simulink model "simulation"  (R2020a)
settings: Solver=VariableStepAuto  StartTime=0.0  StopTime=50  RelTol=1e-3
libraries: SignalEditorBlockLib x3
settings Model: Creator=MILAD  LastModifiedBy=payagostar
settings DataIOCC: ReturnWorkspaceOutputs=off
settings DebuggingCC: ArithmeticOperatorsInVariantConditions=warning
settings SFSimCC: CustomCodeUndefinedFunction=UseInterfaceOnly

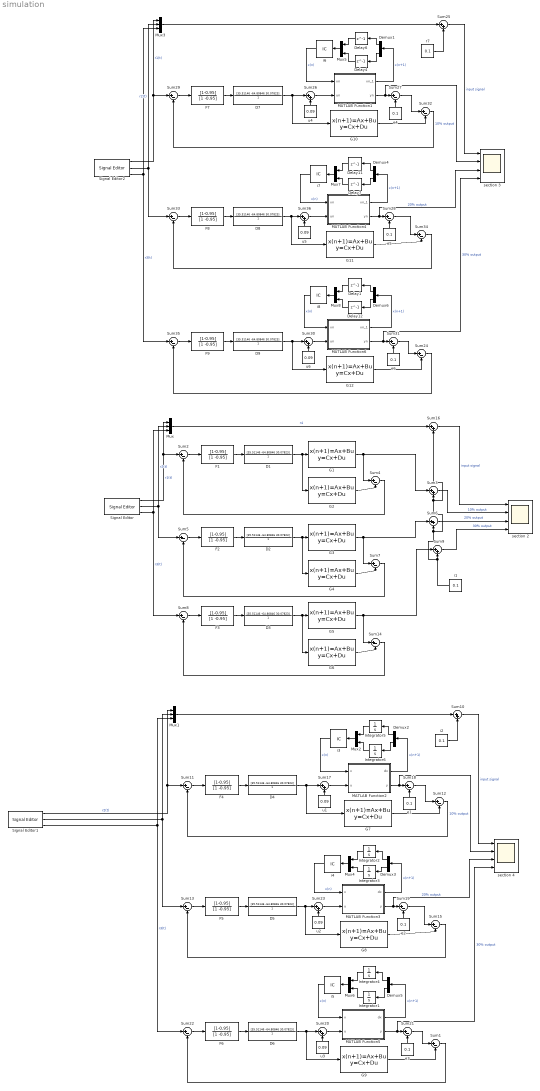
== system simulation ==
  " section 2" : Scope  NumInputPorts=4
  D{1..9} (9 alike) : DiscreteFilter  Numerator=[35.51146 -64.80846 30.07823]  Denominator=1  SampleTime=0.166
  Delay{1,4,6..7,11..12} (6 alike) : Delay  DelayLength=1  InitialCondition=0  SampleTime=0.166
  Demux{1..6} (6 alike) : Demux  Outputs=2
  F{1..9} (9 alike) : DiscreteFilter  Numerator=[1-0.95]  Denominator=[1 -0.95]  SampleTime=0.166
  G{1..12} (12 alike) : DiscreteStateSpace  A=[0.9884 0.1523;-0.1354 0.8361]  B=[0.01447;0.1693]  C=[1 0]  D=0  SampleTime=0.166
  Integrator1 : Integrator
  Integrator2 : Integrator  InitialCondition=0.1
  Integrator3 : Integrator
  Integrator4 : Integrator  InitialCondition=0.1
  Integrator5 : Integrator  InitialCondition=0.1
  Integrator6 : Integrator
  MATLAB Function1 : MATLAB Function  TreatAsAtomicUnit=on
  MATLAB Function2 : MATLAB Function  TreatAsAtomicUnit=on
  MATLAB Function3 : MATLAB Function  TreatAsAtomicUnit=on
  MATLAB Function4 : MATLAB Function  TreatAsAtomicUnit=on
  MATLAB Function5 : MATLAB Function  TreatAsAtomicUnit=on
  MATLAB Function6 : MATLAB Function  TreatAsAtomicUnit=on
  Mux : Mux  Inputs=3
  Mux1 : Mux  Inputs=3
  Mux{2,4..8} (6 alike) : Mux  Inputs=2
  Mux3 : Mux  Inputs=3
  Signal Editor : SignalEditorBlockLib/Signal Editor  FileName=r.mat  ActiveScenario=signal  ActiveSignal=Signal 3  IsBus=off  OutputBusObjectStr=Bus: BusObject  SampleTime=0.166  Interpolate=off  ZeroCross=off  OutputAfterFinalValue=Setting to zero  Unit=inherit  PreserveSignalName=on
  Signal Editor1 : SignalEditorBlockLib/Signal Editor  FileName=r.mat  ActiveScenario=signal  ActiveSignal=Signal 3  IsBus=off  OutputBusObjectStr=Bus: BusObject  SampleTime=0.166  Interpolate=off  ZeroCross=off  OutputAfterFinalValue=Setting to zero  Unit=inherit  PreserveSignalName=on
  Signal Editor2 : SignalEditorBlockLib/Signal Editor  FileName=r.mat  ActiveScenario=signal  ActiveSignal=Signal 3  IsBus=off  OutputBusObjectStr=Bus: BusObject  SampleTime=0.166  Interpolate=off  ZeroCross=off  OutputAfterFinalValue=Setting to zero  Unit=inherit  PreserveSignalName=on
  Sum{1..2,4..5,7..8,11..15,18..19,21..22,24,27..29,31..35} (24 alike) : Sum  Inputs=|+-
  Sum{3,6,9..10,16..17,20,23,25..26,30,36} (12 alike) : Sum  Inputs=|++
  e{1..6} (6 alike) : Constant  Value=0.1  SampleTime=0.166
  i1 : Constant  Value=0.1  SampleTime=0.166
  i2 : Constant  Value=0.1  SampleTime=0.166
  i{3..8} (6 alike) : InitialCondition  Value=[0.1;0]
  r7 : Constant  Value=0.1  SampleTime=0.166
  section 3 : Scope  NumInputPorts=4
  section 4 : Scope  NumInputPorts=4
  u{1..6} (6 alike) : Constant  Value=0.09  SampleTime=0.166
  wires:
  G2/1 -> Sum4/2
  G1/1 -> Sum3/1, Sum4/1
  D1/1 -> G2/1, G1/1
  F1/1 -> D1/1
  Sum2/1 -> F1/1
  Sum4/1 -> Sum2/2
  Signal Editor/1 -> Mux/1, Sum2/1  "r1(t)"
  Sum7/1 -> Sum5/2
  F2/1 -> D2/1
  Sum5/1 -> F2/1
  D2/1 -> G4/1, G3/1
  Signal Editor/2 -> Mux/2, Sum5/1  "r2(t)"
  G3/1 -> Sum6/1, Sum7/1
  G4/1 -> Sum7/2
  Sum14/1 -> Sum8/2
  D3/1 -> G6/1, G5/1
  Signal Editor/3 -> Sum8/1, Mux/3  "r3(t)"
  G5/1 -> Sum9/1, Sum14/1
  G6/1 -> Sum14/2
  i1/1 -> Sum16/2, Sum3/2, Sum6/2, Sum9/2
  Sum3/1 -> " section 2"/2  "10% output"
  Sum6/1 -> " section 2"/3  "20% output"
  Sum9/1 -> " section 2"/4  "30% output"
  Mux/1 -> Sum16/1  "r4"
  Sum16/1 -> " section 2"/1  "input signal"
  F3/1 -> D3/1
  Sum8/1 -> F3/1
  Sum21/1 -> Sum1/1
  Sum23/1 -> MATLAB Function3/2(u)
  e3/1 -> Sum21/2
  Demux3/1 -> Integrator2/1
  i5/1 -> MATLAB Function5/1(x)  "x(n)"
  Mux6/1 -> i5/1
  MATLAB Function5/1(dx) -> Demux5/1  "x(n+1)"
  MATLAB Function5/2(y) -> section 4/4, Sum21/1  "30% output"
  F6/1 -> D6/1
  Sum19/1 -> Sum15/1
  Integrator2/1 -> Mux4/1
  Demux5/1 -> Integrator4/1
  Sum12/1 -> Sum11/2
  Signal Editor1/1 -> Mux1/1, Sum11/1  "r2(t)"
  Sum18/1 -> Sum12/1
  Demux3/2 -> Integrator3/1
  MATLAB Function3/2(y) -> section 4/3, Sum19/1  "20% output"
  e2/1 -> Sum19/2
  Integrator3/1 -> Mux4/2
  Integrator4/1 -> Mux6/1
  Integrator1/1 -> Mux6/2
  u3/1 -> Sum20/2
  Demux2/1 -> Integrator5/1
  u2/1 -> Sum23/2
  Mux4/1 -> i4/1
  Sum17/1 -> MATLAB Function2/2(u)
  D5/1 -> Sum23/1, G8/1
  G9/1 -> Sum1/2
  i2/1 -> Sum10/2
  i4/1 -> MATLAB Function3/1(x)  "x(n)"
  e1/1 -> Sum18/2
  Demux2/2 -> Integrator6/1
  Sum15/1 -> Sum13/2
  Sum10/1 -> section 4/1  "input signal"
  G7/1 -> Sum12/2
  MATLAB Function2/2(y) -> section 4/2, Sum18/1  "10% output"
  Sum22/1 -> F6/1
  Mux1/1 -> Sum10/1
  Sum13/1 -> F5/1
  MATLAB Function3/1(dx) -> Demux3/1  "x(n+1)"
  F5/1 -> D5/1
  Sum20/1 -> MATLAB Function5/2(u)
  MATLAB Function2/1(dx) -> Demux2/1  "x(n+1)"
  Mux2/1 -> i3/1
  u1/1 -> Sum17/2
  Sum1/1 -> Sum22/2
  Integrator5/1 -> Mux2/1
  Sum11/1 -> F4/1
  Integrator6/1 -> Mux2/2
  i3/1 -> MATLAB Function2/1(x)  "x(n)"
  D4/1 -> G7/1, Sum17/1
  Signal Editor1/3 -> Sum22/1, Mux1/3  "r3(t)"
  Signal Editor1/2 -> Sum13/1, Mux1/2
  G8/1 -> Sum15/2
  D6/1 -> Sum20/1, G9/1
  F4/1 -> D4/1
  Demux5/2 -> Integrator1/1
  Sum31/1 -> Sum24/1
  Sum36/1 -> MATLAB Function4/2(un)
  e6/1 -> Sum31/2
  Demux4/1 -> Delay11/1
  i8/1 -> MATLAB Function6/1(xn)  "x(n)"
  Mux8/1 -> i8/1
  MATLAB Function6/1(xn_1) -> Demux6/1  "x(n+1)"
  MATLAB Function6/2(yn) -> section 3/4, Sum31/1  "30% output"
  F9/1 -> D9/1
  Sum28/1 -> Sum34/1
  Delay11/1 -> Mux7/1
  Demux6/1 -> Delay1/1
  Sum32/1 -> Sum29/2
  Signal Editor2/1 -> Mux3/1, Sum29/1  "r1(t)"
  Sum27/1 -> Sum32/1
  Demux4/2 -> Delay7/1
  MATLAB Function4/2(yn) -> section 3/3, Sum28/1  "20% output"
  e5/1 -> Sum28/2
  Delay7/1 -> Mux7/2
  Delay1/1 -> Mux8/1
  Delay12/1 -> Mux8/2
  u6/1 -> Sum30/2
  Demux1/1 -> Delay6/1
  u5/1 -> Sum36/2
  Mux7/1 -> i7/1
  Sum26/1 -> MATLAB Function1/2(un)
  D8/1 -> Sum36/1, G11/1
  G12/1 -> Sum24/2
  r7/1 -> Sum25/2
  i7/1 -> MATLAB Function4/1(xn)  "x(n)"
  e4/1 -> Sum27/2
  Demux1/2 -> Delay4/1
  Sum34/1 -> Sum33/2
  Sum25/1 -> section 3/1  "input signal"
  G10/1 -> Sum32/2
  MATLAB Function1/2(yn) -> section 3/2, Sum27/1  "10% output"
  Sum35/1 -> F9/1
  Mux3/1 -> Sum25/1
  Sum33/1 -> F8/1
  MATLAB Function4/1(xn_1) -> Demux4/1  "x(n+1)"
  F8/1 -> D8/1
  Sum30/1 -> MATLAB Function6/2(un)
  MATLAB Function1/1(xn_1) -> Demux1/1  "x(n+1)"
  Mux5/1 -> i6/1
  u4/1 -> Sum26/2
  Sum24/1 -> Sum35/2
  Delay6/1 -> Mux5/1
  Sum29/1 -> F7/1
  Delay4/1 -> Mux5/2
  i6/1 -> MATLAB Function1/1(xn)  "x(n)"
  D7/1 -> G10/1, Sum26/1
  Signal Editor2/3 -> Mux3/3, Sum35/1  "r3(t)"
  Signal Editor2/2 -> Mux3/2, Sum33/1  "r2(t)"
  G11/1 -> Sum34/2
  D9/1 -> Sum30/1, G12/1
  F7/1 -> D7/1
  Demux6/2 -> Delay12/1

== matlab function simulation/MATLAB Function4 ==
  data: xn input; xn_1 output; un input; yn output
function [xn_1,yn] = g1(xn,un)
xn_1 = [xn(1)+0.166*xn(2);-0.166*xn(1)+(1-0.166)*xn(2)+0.166*un/(1-xn(1))];
yn = [1 0]*xn;

== matlab function simulation/MATLAB Function2 ==
  data: x input; dx output; u input; y output
function [dx,y] = System(x,u)
dx = [x(2);-x(1)-x(2)+u/(1-x(1))];
y  = [1 0]*x;

== matlab function simulation/MATLAB Function3 ==
  data: x input; dx output; u input; y output
function [dx,y] = System(x,u)
dx = [x(2);-x(1)-x(2)+u/(1-x(1))];
y  = [1 0]*x;

== matlab function simulation/MATLAB Function6 ==
  data: xn input; xn_1 output; un input; yn output
function [xn_1,yn] = g1(xn,un)
xn_1 = [xn(1)+0.166*xn(2);-0.166*xn(1)+(1-0.166)*xn(2)+0.166*un/(1-xn(1))];
yn = [1 0]*xn;

== matlab function simulation/MATLAB Function5 ==
  data: x input; dx output; u input; y output
function [dx,y] = System(x,u)
dx = [x(2);-x(1)-x(2)+u/(1-x(1))];
y  = [1 0]*x;

== matlab function simulation/MATLAB Function1 ==
  data: xn input; xn_1 output; un input; yn output
function [xn_1,yn] = g1(xn,un)
xn_1 = [xn(1)+0.166*xn(2);-0.166*xn(1)+(1-0.166)*xn(2)+0.166*un/(1-xn(1))];
yn = [1 0]*xn;
